simulink model "Decoder3_8"  (R2025b)
settings: Solver=VariableStepAuto  StartTime=0.0  StopTime=10.0  RelTol=1e-3
settings Model: Creator=sjpau  LastModifiedBy=Johan

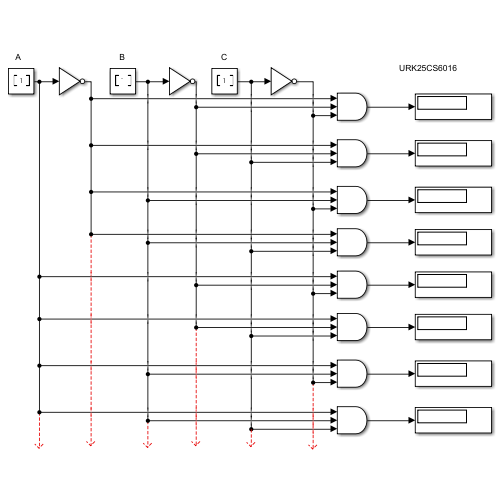
[thumbnail: Simulink's stored preview of the top-level diagram]
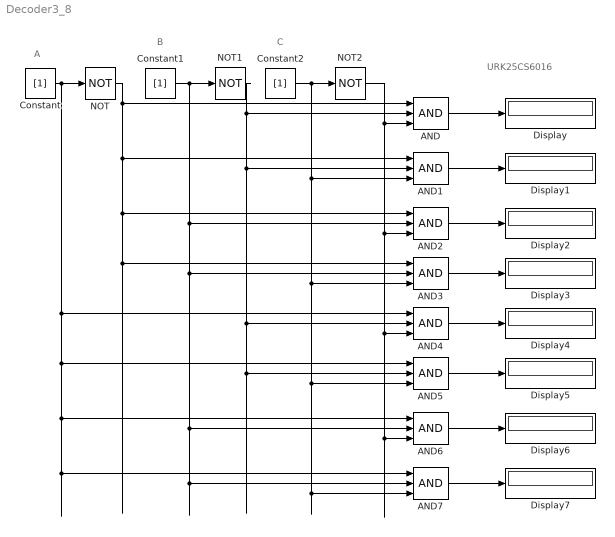
== system Decoder3_8 ==
  note: URK25CS6016
  note: C
  note: B
  note: A
  AND{,1..7} (8 alike) : Logic  Inputs=3  IconShape=distinctive  AllPortsSameDT=off  OutDataTypeStr=boolean
  Constant : Constant  Value=[1]
  Constant1 : Constant  Value=[1]
  Constant2 : Constant  Value=[1]
  Display{,1..7} (8 alike) : Display
  NOT : Logic  Operator=NOT  IconShape=distinctive  AllPortsSameDT=off  OutDataTypeStr=boolean
  NOT1 : Logic  Operator=NOT  IconShape=distinctive  AllPortsSameDT=off  OutDataTypeStr=boolean
  NOT2 : Logic  Operator=NOT  IconShape=distinctive  AllPortsSameDT=off  OutDataTypeStr=boolean
  wires:
  Constant/1 -> AND5/1, AND6/1, AND7/1, AND4/1, NOT/1
  Constant1/1 -> NOT1/1, AND3/2, AND6/2, AND7/2, AND2/2
  Constant2/1 -> NOT2/1, AND3/3, AND5/3, AND7/3, AND1/3
  NOT/1 -> AND2/1, AND3/1, AND1/1, AND/1
  NOT1/1 -> AND1/2, AND4/2, AND5/2, AND/2
  NOT2/1 -> AND6/3, AND4/3, AND2/3, AND/3
  AND/1 -> Display/1
  AND1/1 -> Display1/1
  AND2/1 -> Display2/1
  AND3/1 -> Display3/1
  AND4/1 -> Display4/1
  AND5/1 -> Display5/1
  AND6/1 -> Display6/1
  AND7/1 -> Display7/1
